simulink model "model2v3"  (R2020b)
settings: Solver=VariableStepAuto  StartTime=0.0  StopTime=10.0  RelTol=1e-3
settings Model: Creator=dkravchenko  LastModifiedBy=dkravchenko

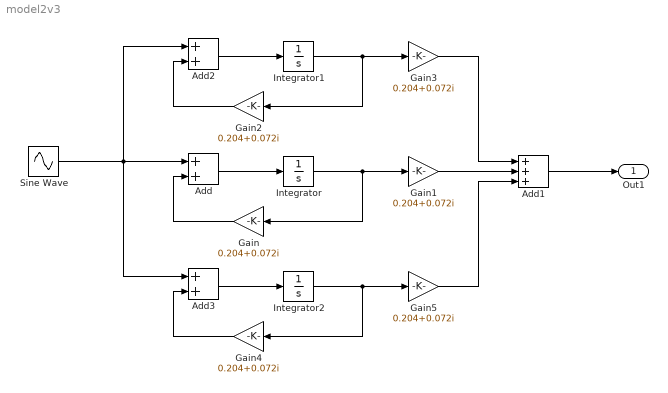
== system model2v3 ==
  Add : Sum
  Add1 : Sum  Inputs=+++
  Add2 : Sum
  Add3 : Sum
  Gain{,1..5} (6 alike) : Gain  Gain=0.204+0.072i
  Integrator : Integrator
  Integrator1 : Integrator
  Integrator2 : Integrator
  Sine Wave : Sin  SampleTime=0
  Out1 : Outport
  wires:
  Add/1 -> Integrator/1
  Integrator/1 -> Gain1/1, Gain/1
  Gain/1 -> Add/2
  Gain1/1 -> Add1/2
  Add1/1 -> Out1/1
  Integrator1/1 -> Gain3/1, Gain2/1
  Gain2/1 -> Add2/2
  Add2/1 -> Integrator1/1
  Gain3/1 -> Add1/1
  Sine Wave/1 -> Add3/1, Add2/1, Add/1
  Integrator2/1 -> Gain5/1, Gain4/1
  Gain4/1 -> Add3/2
  Add3/1 -> Integrator2/1
  Gain5/1 -> Add1/3
